simulink subsystem "BatteryHV_input_refsub"  (R2022a)
settings: Solver=VariableStepAuto  StartTime=0.0  StopTime=10.0  RelTol=1e-3
settings Model: Creator=isaacito  LastModifiedBy=isaacito

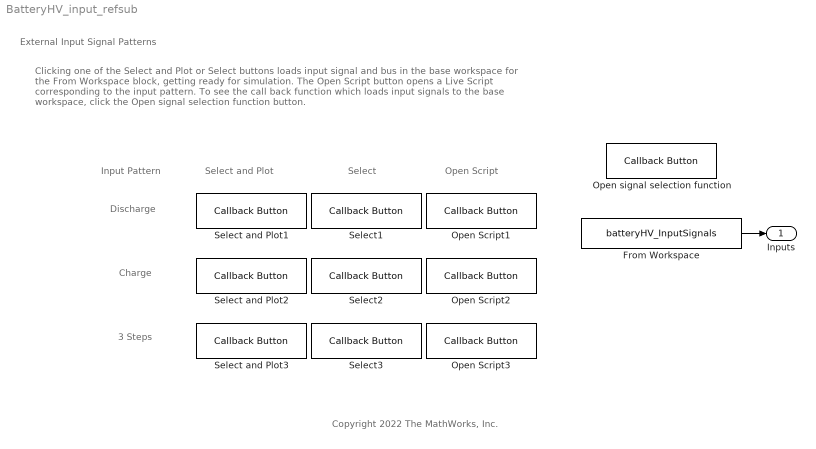
== system BatteryHV_input_refsub ==
  note: Clicking one of the Select and Plot or Select buttons loads input signal and bus
      | in the base workspace for the From Workspace block, getting ready for simulation.
      | The Open Script button opens a Live Script corresponding to the input pattern.
      | To see the call back function which loads input signals to the base workspace,
      | click the Open signal selection function button.
  note: Select
  note: Input Pattern
  note: Open Script
  note: Discharge
  note: Select and Plot
  note: External Input Signal Patterns
  note: Copyright 2022 The MathWorks, Inc.
  note: Charge
  note: 3 Steps
  From Workspace : FromWorkspace  VariableName=batteryHV_InputSignals  OutDataTypeStr=Bus: batteryHV_InputBus  OutputAfterFinalValue=Holding final value
      settings: AttributesFormatString=|
      | %<OutDataTypeStr>
      | Interpolate: %<Interpolate>
  Open Script1 : CallbackButton  ButtonText=Open Script
      settings: ClickFcn=edit BatteryHV_testcase_Discharge
  Open Script2 : CallbackButton  ButtonText=Open Script
      settings: ClickFcn=edit BatteryHV_testcase_Charge
  Open Script3 : CallbackButton  ButtonText=Open Script
      settings: ClickFcn=edit BatteryHV_testcase_LoadCurrentStep3
  Open signal selection function : CallbackButton  ButtonText=Open function
      settings: ClickFcn=edit BatteryHV_selectInput
  Select and Plot1 : CallbackButton  ButtonText=Select and Plot
      settings: ClickFcn=|
      | BatteryHV_selectInput( ...
      |     InputPattern = "Discharge", ...
      |     DisplayMessage = true )
      | 
      | BatteryHV_plotInputs( ...
      |     "batteryHV_InputSignals", ...
      |     WindowName = "Discharge");
  Select and Plot2 : CallbackButton  ButtonText=Select and Plot
      settings: ClickFcn=|
      | BatteryHV_selectInput( ...
      |     InputPattern = "Charge", ...
      |     DisplayMessage = true )
      | 
      | BatteryHV_plotInputs( ...
      |     "batteryHV_InputSignals", ...
      |     WindowName = "Charge");
  Select and Plot3 : CallbackButton  ButtonText=Select and Plot
      settings: ClickFcn=|
      | BatteryHV_selectInput( ...
      |     InputPattern = "LoadCurrentStep3", ...
      |     DisplayMessage = true )
      | 
      | BatteryHV_plotInputs( ...
      |     "batteryHV_InputSignals", ...
      |     WindowName = "LoadCurrentStep3");
  Select1 : CallbackButton  ButtonText=Select
      settings: ClickFcn=|
      | BatteryHV_selectInput( ...
      |     InputPattern = "Discharge", ...
      |     DisplayMessage = true )
  Select2 : CallbackButton  ButtonText=Select
      settings: ClickFcn=|
      | BatteryHV_selectInput( ...
      |     InputPattern = "Charge", ...
      |     DisplayMessage = true )
  Select3 : CallbackButton  ButtonText=Select
      settings: ClickFcn=|
      | BatteryHV_selectInput( ...
      |     InputPattern = "LoadCurrentStep3", ...
      |     DisplayMessage = true )
  Inputs : Outport
  wires:
  From Workspace/1 -> Inputs/1
